simulink model "assgn1a"  (R2021a)
settings: Solver=VariableStepAuto  StartTime=0.0  StopTime=10.0  RelTol=1e-3
values from neighbouring files (symbols this model uses):
  c1 = 100    [assgn1_cnst.m]
  c2 = 1000    [assgn1_cnst.m]
  k1 = 1e4    (= 10000)    [assgn1_cnst.m]
  k2 = 1e5    (= 100000)    [assgn1_cnst.m]
  m1 = 10    [assgn1_cnst.m]
  m2 = 100    [assgn1_cnst.m]
settings Model: Creator=shrutidalal  LastModifiedBy=shrutidalal

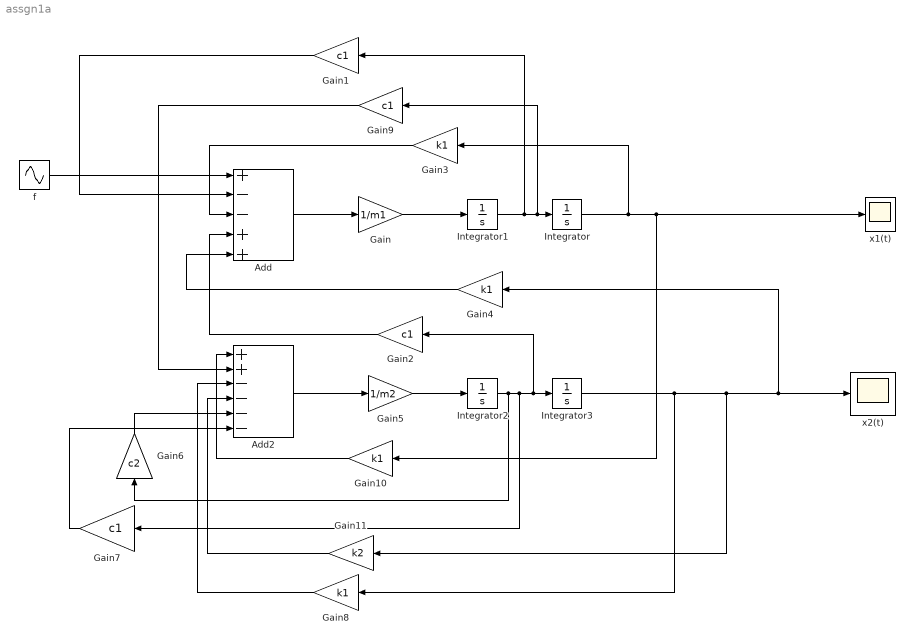
== system assgn1a ==
  Add : Sum  Inputs=+--++
  Add2 : Sum  Inputs=++----
  Gain : Gain  Gain=1/m1
  Gain{1..2,7,9} (4 alike) : Gain  Gain=c1
  Gain{3..4,8,10} (4 alike) : Gain  Gain=k1
  Gain11 : Gain  Gain=k2
  Gain5 : Gain  Gain=1/m2
  Gain6 : Gain  Gain=c2
  Integrator{,1..3} (4 alike) : Integrator
  f : Sin  SampleTime=0
  x1(t) : Scope
  x2(t) : Scope
  wires:
  Gain11/1 -> Add2/4
  Gain9/1 -> Add2/2
  Gain2/1 -> Add/4
  Gain6/1 -> Add2/5
  Gain8/1 -> Add2/3
  Add/1 -> Gain/1
  Integrator3/1 -> Gain8/1, Gain11/1, x2(t)/1, Gain4/1
  Gain1/1 -> Add/2
  Gain4/1 -> Add/5
  Gain5/1 -> Integrator2/1
  Add2/1 -> Gain5/1
  Integrator/1 -> Gain3/1, Gain10/1, x1(t)/1
  Integrator2/1 -> Gain6/1, Gain7/1, Gain2/1, Integrator3/1
  Gain3/1 -> Add/3
  Gain7/1 -> Add2/6
  Gain10/1 -> Add2/1
  Integrator1/1 -> Gain1/1, Gain9/1, Integrator/1
  f/1 -> Add/1
  Gain/1 -> Integrator1/1
